simulink model "CodeMATLAB"  (R2020a)
settings: Solver=ode8  StartTime=0.0  StopTime=inf  FixedStep=0.05  RelTol=1e-3
PreLoadFcn:
  | waijung.modelPreload; % Required for working with Waijung Blockset. Do not remove.
undefined symbols (not defined in the file): Blocking, DiscIntNeverNeededParam, HSEOSC, LF, Link, LQFP100, Non, ST, STM32F407VG
libraries: amg_usbconverter_n_connect_lib x3, stm32f4_io_lib x2, simulink x2, stm32f4_tim_lib x1, stm32f4_reset_lib x1, stm32f4_device_config_lib x1
CloseFcn:
  | waijung.modelClose; % Required for working with Waijung Blockset. Do not remove.
settings Model: EnablePacing=on  Creator=tanda  LastModifiedBy=tanda
settings OptimizationCC: DefaultParameterBehavior=Inlined  EnhancedBackFolding=on  PassReuseOutputArgsAs=Individual arguments  ZeroExternalMemoryAtStartup=off  ZeroInternalMemoryAtStartup=off  OptimizeBlockOrder=speed  DifferentSizesBufferReuse=on  OptimizationCustomize=off  EfficientTunableParamExpr=on
settings DebuggingCC: ParameterTunabilityLossMsg=error
settings HardwareCC: ProdBitPerPointer=32  ProdBitPerSizeT=32  ProdBitPerPtrDiffT=32  ProdLargestAtomicFloat=None  ProdIntDivRoundTo=Undefined  ProdWordSize=32  ProdHWDeviceType=ARM Compatible->Cortex - M4  TargetEndianess=LittleEndian  TargetHWDeviceType=ARM Compatible->Cortex - M4
settings SFSimCC: MATLABDynamicMemAlloc=off
settings RTWCC: Description=STM32F4 Target  SystemTargetFile=stm32f4.tlc  GenerateMakefile=off  TemplateMakefile=ert_default_tmf
settings CodeAppCC: ForceParamTrailComments=on  IgnoreCustomStorageClasses=off  OperatorAnnotations=on  SimulinkDataObjDesc=on  SFDataObjDesc=on  InsertBlockDesc=on
settings STFCustomTargetCC: TargetLangStandard=C99 (ISO)  MultiwordLength=256  ModelReferenceCompliant=off  CombineOutputUpdateFcns=on  ERTCustomFileBanners=on  SupportContinuousTime=off  SupportNonInlinedSFcns=off  RemoveResetFunc=on  MATLABClassNameForMDSCustomization=Simulink.SoftwareTarget.ERTCustomization  SystemTargetFile=stm32f4.tlc
settings ERTTargetCC: TargetLangStandard=C99 (ISO)  ModelReferenceCompliant=off  ParMdlRefBuildCompliant=off  CompOptLevelCompliant=off  ConcurrentExecutionCompliant=off  ModelStepFunctionPrototypeControlCompliant=off  CPPClassGenCompliant=off  UseToolchainInfoCompliant=off  InlinedParameterPlacement=NonHierarchical  ERTSrcFileBannerTemplate=stm32f4_code_template.cgt  ERTHdrFileBannerTemplate=stm32f4_code_template.cgt  ERTDataSrcFileTemplate=stm32f4_code_template.cgt  ERTDataHdrFileTemplate=stm32f4_code_template.cgt  ERTCustomFileTemplate=stm32f4_file_process.tlc

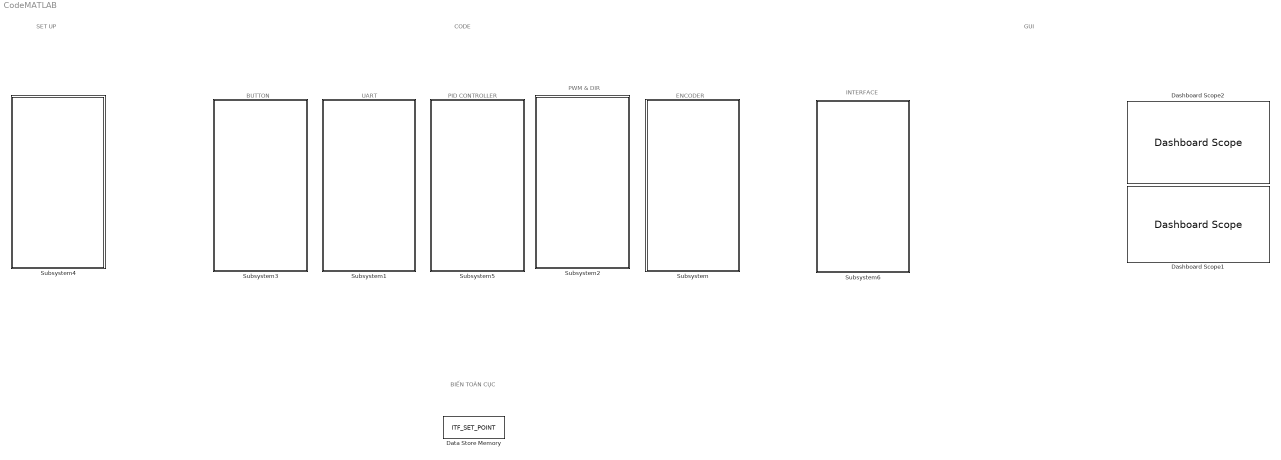
== system CodeMATLAB ==
  note: ENCODER
  note: SET UP
  note: CODE
  note: UART
  note: PWM & DIR
  note: BUTTON
  note: PID CONTROLLER
  note: INTERFACE
  note: GUI
  note: BIẾN TOÀN CỤC
  Dashboard Scope1 : DashboardScope
  Dashboard Scope2 : DashboardScope
  Data Store Memory : DataStoreMemory  DataStoreName=ITF_SET_POINT  ReadBeforeWriteMsg=warning  WriteAfterWriteMsg=warning  WriteAfterReadMsg=warning  ShowAdditionalParam=off  OutMin=-800  OutMax=800
      settings: DataLoggingMaxPoints=800
  Subsystem : Subsystem
  Subsystem1 : Subsystem
  Subsystem2 : Subsystem
  Subsystem3 : Subsystem
  Subsystem4 : Subsystem
  Subsystem5 : Subsystem
  Subsystem6 : Subsystem
  wires:
  ? -> ?

== system CodeMATLAB/Subsystem ==
  Doc encoder : Subsystem  TreatAsAtomicUnit=on
  Rate Transition2 : RateTransition  Deterministic=off  OutPortSampleTime=0.05
  Timer (Time Base) IRQ : stm32f4_tim_lib/Timer (Time Base) IRQ  configmode=Advance  timer=9  nvicprioritygroup=4  irqpreemptionpriority_g0=0  irqpreemptionpriority_g1=0  irqpreemptionpriority_g2=0  irqpreemptionpriority_g3=0  irqpreemptionpriority_g4=0  irqpreemptionpriority=0  irqsubpriority_g0=0  irqsubpriority_g1=0  irqsubpriority_g2=0  irqsubpriority_g3=0  irqsubpriority_g4=0  irqsubpriority=0  sampletime=0.05  autoreload=65115  prescaler=128  blockid=SubsystemTimerTimeBaseIRQ
      settings: SourceProductName=Waijung Blockset
  tag scope: SPEED=global
  wires:
  Doc encoder/1(Speed) -> Rate Transition2/1
  Timer (Time Base) IRQ/1 -> Doc encoder/Trigger
  Rate Transition2/1 -> [SPEED]

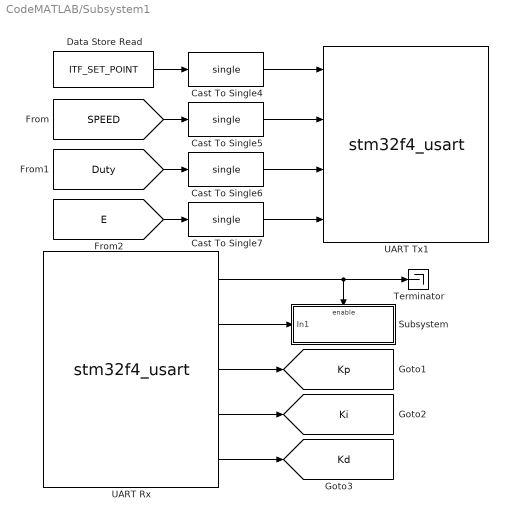
== system CodeMATLAB/Subsystem1 ==
  Cast To Single{4..7} (4 alike) : DataTypeConversion  OutDataTypeStr=single
  Data Store Read : DataStoreRead  DataStoreName=ITF_SET_POINT  DataStoreElements=ITF_SET_POINT
  Subsystem : Subsystem
  Terminator : Terminator
  UART Rx : S-Function  Priority=1  FunctionName=stm32f4_usart  Parameters=configuration,uartmodule,transfer,baudrate,inputtype,outputtype,confstr,binheaderarray,binterminatorarray,asciiheader,asciiterminator,bindatalength,packetmode,varname,sampletime,sampletimestr,blockid  SFunctionDeploymentMode=off  EnableBusSupport=off  mask(stm32f4_usart){configuration=Rx, uartmodule=6, baudrate=115200, databits=8, parity=No, stopbit=1, remaptxpin=Not used, remaprxpin=Not used, flowcontrol=None, remapctspin=Not used, remaprtspin=Not used, advanceoptions=off, rxbuffersize=512, txbuffersize=512, transfer=Non-Blocking, packetmode=Ascii, binheader='53', binterminator='00', porttype_double=0, porttype_single=0, porttype_int8=0, porttype_uint8=0, porttype_int16=0, porttype_uint16=0, porttype_int32=0, porttype_uint32=0, asciiformat='%f,%f,%f,%f', rx_asciiterminator=LF (0x0A - "\n"), tx_asciiterminator=LF (0x0A - "\n"), storagename=<empty>, varname=, inputtype=[0], outputtype=[5 3  1 1 1 1], binheaderarray=[0], binterminatorarray=[0], bindatalength=0, asciiheader='%f,%f,%f,%f\n', asciiterminator=[1 10], sampletime=-1, sampletimestr=-1, blockid=Subsystem1UARTRx, confstr=[ "dummy", "0", "*", "*", "0", "*", "*", "0", "*", "*", "0", "*", "*", "2", "5", "6", "2", "5", "1", "512", "512", "2", "6", "115200", "8", "No", "1", "None", "USART6"], lastmodule=1}
      mask prompts: uartmodule "UART Module"; baudrate "Baud rate (bps)"; databits "Data bits"; stopbit "Stop bit"; remaptxpin "Tx Pin"; remaprxpin "Rx Pin"; flowcontrol "Hardware flow control"; remapctspin "HW Flow control, CTS Pin"; remaprtspin "HW Flow control, RTS Pin"; advanceoptions "Advance options"; rxbuffersize "Rx buffer size (bytes)"; txbuffersize "Tx buffer size (bytes)"; packetmode "Packet mode"; binheader "Binary header (example: '7E 7E')"; binterminator "Binary terminator (example: '03 03')"; porttype_double "Number of data port, type DOUBLE"; porttype_single "Number of data port, type SINGLE"; porttype_int8 "Number of data port, type INT8"; porttype_uint8 "Number of data port, type UINT8"; porttype_int16 "Number of data port, type INT16"; porttype_uint16 "Number of data port, type UINT16"; porttype_int32 "Number of data port, type INT32"; porttype_uint32 "Number of data port, type UINT32"; asciiformat "Ascii format"; rx_asciiterminator "End of packet"; tx_asciiterminator "End of packet"; storagename "Buffer"; varname "Var name"; inputtype "Input data type"; outputtype "Output data type"; binheaderarray "Binary header"; binterminatorarray "Binary terminator"; bindatalength "Binary data length"; asciiheader "Ascii header (printf format)"; asciiterminator "Ascii terminator"; sampletime "Sample time (sec)"; sampletimestr "Compiled sample time (sec) in string"; confstr "Configuration string"; lastmodule "Last module selected"
      mask help:
      | Data type for Ascii format
      | %u, %i, %d, %o, %x: uint32
      | %e, %g, %f: single
      | %c: int8
      mask init:
      | stm32f4_usart_callback('init');
      mask Help: web(fullfile(waijungdocroot,'stm32f4_usart_rx.htm'), '-browser')
      mask TypeOptions configuration: Setup | Tx | Rx
      mask Callback configuration: stm32f4_usart_callback('configuration');
      mask TypeOptions uartmodule: 1 | 2 | 3 | 4 | 5 | 6
      mask Callback uartmodule: stm32f4_usart_callback('uartmodule');
      mask Callback baudrate: stm32f4_usart_callback('baudrate');
      mask TypeOptions databits: 8
      mask TypeOptions parity: No | Odd | Even
      mask TypeOptions stopbit: 0.5 | 1 | 1.5 | 2
      mask TypeOptions remaptxpin: Not used | A9 | B6
      mask TypeOptions remaprxpin: Not used | A10 | B7
      mask TypeOptions flowcontrol: None | RTS | CTS | RTS/CTS
      mask Callback flowcontrol: stm32f4_usart_callback('flowcontrol');
      mask TypeOptions remapctspin: Not used | A11
      mask TypeOptions remaprtspin: Not used | A12
      mask Callback advanceoptions: stm32f4_usart_callback('advanceoptions');
      mask TypeOptions rxbuffersize: 16 | 32 | 64 | 128 | 256 | 512 | 1024 | 2048
      mask TypeOptions txbuffersize: 16 | 32 | 64 | 128 | 256 | 512 | 1024 | 2048
      mask TypeOptions transfer: Blocking | Non-Blocking
      mask Callback transfer: stm32f4_usart_callback('transfer');
      mask TypeOptions packetmode: Ascii | Binary | Binary Vector | String Buffer | Raw Buffer | Read Line
      mask Callback packetmode: stm32f4_usart_callback('packetmode');
      mask Callback binheader: stm32f4_usart_callback('binheader');
      mask Callback binterminator: stm32f4_usart_callback('binterminator');
      mask Callback porttype_double: stm32f4_usart_callback('porttype');
      mask Callback porttype_single: stm32f4_usart_callback('porttype');
      mask Callback porttype_int8: stm32f4_usart_callback('porttype');
      mask Callback porttype_uint8: stm32f4_usart_callback('porttype');
      mask Callback porttype_int16: stm32f4_usart_callback('porttype');
      mask Callback porttype_uint16: stm32f4_usart_callback('porttype');
      mask Callback porttype_int32: stm32f4_usart_callback('porttype');
      mask Callback porttype_uint32: stm32f4_usart_callback('porttype');
      mask Callback asciiformat: stm32f4_usart_callback('asciiformat');
      mask TypeOptions rx_asciiterminator: CR (0x0D - "\r") | LF (0x0A - "\n") | CRLF (0x0D 0x0A - "\r\n")
      mask Callback rx_asciiterminator: stm32f4_usart_callback('rx_asciiterminator');
      mask TypeOptions tx_asciiterminator: CR (0x0D - "\r") | LF (0x0A - "\n") | CRLF (0x0D 0x0A - "\r\n") | None
      mask Callback tx_asciiterminator: stm32f4_usart_callback('tx_asciiterminator');
      mask TypeOptions storagename: <empty>
      mask Callback storagename: stm32f4_usart_callback('storagename');
      mask Callback varname: stm32f4_usart_callback('varname');
      mask Callback sampletime: stm32f4_usart_callback('sampletime');
      mask Callback sampletimestr: stm32f4_usart_callback('sampletimestr');
      mask Callback blockid: stm32f4_usart_callback('blockid');
      mask Display: text(0.05, 0.5, 'Module: USART6_Rx\nPacket: Ascii\nTransfer: Non-Blocking\nTs (sec): -1','ver','middle','hor','left'); port_label('output', 1,'READY'); port_label('output', 2,'single'); port_label('output', 3,'single'); port_label('output', 4,'single'); port_label('output', 5,'single');
  UART Tx1 : S-Function  Priority=1  FunctionName=stm32f4_usart  Parameters=configuration,uartmodule,transfer,baudrate,inputtype,outputtype,confstr,binheaderarray,binterminatorarray,asciiheader,asciiterminator,bindatalength,packetmode,varname,sampletime,sampletimestr,blockid  SFunctionDeploymentMode=off  EnableBusSupport=off  mask(stm32f4_usart){configuration=Tx, uartmodule=6, baudrate=115200, databits=8, parity=No, stopbit=1, remaptxpin=Not used, remaprxpin=Not used, flowcontrol=None, remapctspin=Not used, remaprtspin=Not used, advanceoptions=off, rxbuffersize=512, txbuffersize=512, transfer=Non-Blocking, packetmode=Ascii, binheader='7E 7E', binterminator='03 03', porttype_double=2, porttype_single=0, porttype_int8=0, porttype_uint8=0, porttype_int16=0, porttype_uint16=0, porttype_int32=0, porttype_uint32=0, asciiformat='%f,%f,%f,%f', rx_asciiterminator=CRLF (0x0D 0x0A - "\r\n"), tx_asciiterminator=LF (0x0A - "\n"), storagename=<empty>, varname=, inputtype=[4  1 1 1 1], outputtype=[0], binheaderarray=[0], binterminatorarray=[0], bindatalength=0, asciiheader='%f,%f,%f,%f\n', asciiterminator=[1 10], sampletime=0.05, sampletimestr=-1, blockid=Subsystem1UARTTx1, confstr=[ "dummy", "0", "*", "*", "0", "*", "*", "0", "*", "*", "0", "*", "*", "2", "5", "6", "2", "5", "1", "512", "512", "2", "6", "115200", "8", "No", "1", "None", "USART6"], lastmodule=1}
      mask prompts: uartmodule "UART Module"; baudrate "Baud rate (bps)"; databits "Data bits"; stopbit "Stop bit"; remaptxpin "Tx Pin"; remaprxpin "Rx Pin"; flowcontrol "Hardware flow control"; remapctspin "HW Flow control, CTS Pin"; remaprtspin "HW Flow control, RTS Pin"; advanceoptions "Advance options"; rxbuffersize "Rx buffer size (bytes)"; txbuffersize "Tx buffer size (bytes)"; packetmode "Packet mode"; binheader "Binary header (example: '7E 7E')"; binterminator "Binary terminator (example: '03 03')"; porttype_double "Number of data port, type DOUBLE"; porttype_single "Number of data port, type SINGLE"; porttype_int8 "Number of data port, type INT8"; porttype_uint8 "Number of data port, type UINT8"; porttype_int16 "Number of data port, type INT16"; porttype_uint16 "Number of data port, type UINT16"; porttype_int32 "Number of data port, type INT32"; porttype_uint32 "Number of data port, type UINT32"; asciiformat "Ascii format"; rx_asciiterminator "End of packet"; tx_asciiterminator "End of packet"; storagename "Buffer"; varname "Var name"; inputtype "Input data type"; outputtype "Output data type"; binheaderarray "Binary header"; binterminatorarray "Binary terminator"; bindatalength "Binary data length"; asciiheader "Ascii header (printf format)"; asciiterminator "Ascii terminator"; sampletime "Sample time (sec)"; sampletimestr "Compiled sample time (sec) in string"; confstr "Configuration string"; lastmodule "Last module selected"
      mask help:
      | Data type for Ascii format
      | %u, %i, %d, %o, %x: uint32
      | %e, %g, %f: single
      | %c: int8
      mask init:
      | stm32f4_usart_callback('init');
      mask Help: web(fullfile(waijungdocroot,'stm32f4_usart_tx.htm'), '-browser')
      mask TypeOptions configuration: Setup | Tx | Rx
      mask Callback configuration: stm32f4_usart_callback('configuration');
      mask TypeOptions uartmodule: 1 | 2 | 3 | 4 | 5 | 6
      mask Callback uartmodule: stm32f4_usart_callback('uartmodule');
      mask Callback baudrate: stm32f4_usart_callback('baudrate');
      mask TypeOptions databits: 8
      mask TypeOptions parity: No | Odd | Even
      mask TypeOptions stopbit: 0.5 | 1 | 1.5 | 2
      mask TypeOptions remaptxpin: Not used | A9 | B6
      mask TypeOptions remaprxpin: Not used | A10 | B7
      mask TypeOptions flowcontrol: None | RTS | CTS | RTS/CTS
      mask Callback flowcontrol: stm32f4_usart_callback('flowcontrol');
      mask TypeOptions remapctspin: Not used | A11
      mask TypeOptions remaprtspin: Not used | A12
      mask Callback advanceoptions: stm32f4_usart_callback('advanceoptions');
      mask TypeOptions rxbuffersize: 16 | 32 | 64 | 128 | 256 | 512 | 1024 | 2048
      mask TypeOptions txbuffersize: 16 | 32 | 64 | 128 | 256 | 512 | 1024 | 2048
      mask TypeOptions transfer: Blocking | Non-Blocking
      mask Callback transfer: stm32f4_usart_callback('transfer');
      mask TypeOptions packetmode: Ascii | Binary | Binary Vector | String Buffer | Raw Buffer
      mask Callback packetmode: stm32f4_usart_callback('packetmode');
      mask Callback binheader: stm32f4_usart_callback('binheader');
      mask Callback binterminator: stm32f4_usart_callback('binterminator');
      mask Callback porttype_double: stm32f4_usart_callback('porttype');
      mask Callback porttype_single: stm32f4_usart_callback('porttype');
      mask Callback porttype_int8: stm32f4_usart_callback('porttype');
      mask Callback porttype_uint8: stm32f4_usart_callback('porttype');
      mask Callback porttype_int16: stm32f4_usart_callback('porttype');
      mask Callback porttype_uint16: stm32f4_usart_callback('porttype');
      mask Callback porttype_int32: stm32f4_usart_callback('porttype');
      mask Callback porttype_uint32: stm32f4_usart_callback('porttype');
      mask Callback asciiformat: stm32f4_usart_callback('asciiformat');
      mask TypeOptions rx_asciiterminator: CR (0x0D - "\r") | LF (0x0A - "\n") | CRLF (0x0D 0x0A - "\r\n")
      mask Callback rx_asciiterminator: stm32f4_usart_callback('rx_asciiterminator');
      mask TypeOptions tx_asciiterminator: CR (0x0D - "\r") | LF (0x0A - "\n") | CRLF (0x0D 0x0A - "\r\n") | None
      mask Callback tx_asciiterminator: stm32f4_usart_callback('tx_asciiterminator');
      mask TypeOptions storagename: <empty>
      mask Callback storagename: stm32f4_usart_callback('storagename');
      mask Callback varname: stm32f4_usart_callback('varname');
      mask Callback sampletime: stm32f4_usart_callback('sampletime');
      mask Callback sampletimestr: stm32f4_usart_callback('sampletimestr');
      mask Callback blockid: stm32f4_usart_callback('blockid');
      mask Display: text(0.5, 0.5, 'Module: USART6_Tx\nPacket: Ascii\nTransfer: Non-Blocking\nTs (sec): -1','ver','middle','hor','center'); port_label('input', 1,'single'); port_label('input', 2,'single'); port_label('input', 3,'single'); port_label('input', 4,'single');
  tag scope: Kd=global, Ki=global, Kp=global
  wires:
  UART Rx/1 -> Terminator/1, Subsystem/Enable
  UART Rx/3 -> [Kp]
  UART Rx/4 -> [Ki]
  UART Rx/5 -> [Kd]
  Data Store Read/1 -> Cast To Single4/1
  [SPEED] -> Cast To Single5/1
  [Duty] -> Cast To Single6/1
  [E] -> Cast To Single7/1
  Cast To Single4/1 -> UART Tx1/1
  Cast To Single5/1 -> UART Tx1/2
  Cast To Single6/1 -> UART Tx1/3
  Cast To Single7/1 -> UART Tx1/4
  UART Rx/2 -> Subsystem/1(In1)

== system CodeMATLAB/Subsystem2 ==
  Xuat tin hieu : Subsystem
  wires:
  [Duty] -> Xuat tin hieu/1(Duty)

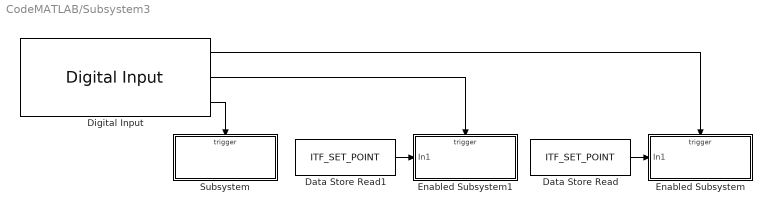
== system CodeMATLAB/Subsystem3 ==
  Data Store Read : DataStoreRead  DataStoreName=ITF_SET_POINT  DataStoreElements=ITF_SET_POINT
  Data Store Read1 : DataStoreRead  DataStoreName=ITF_SET_POINT  DataStoreElements=ITF_SET_POINT
  Digital Input : stm32f4_io_lib/Digital Input  port=D  speed=100  porttype=Pull Down  porttypestr=DOWN  use_pin0=on  use_pin1=off  use_pin2=on  use_pin3=off  use_pin4=on  use_pin5=off  use_pin6=off  use_pin7=off  use_pin8=off  use_pin9=off  use_pin10=off  use_pin11=off  use_pin12=off  use_pin13=off  use_pin14=off  use_pin15=off  pinstr=GPIO_Pin_0 | GPIO_Pin_2 | GPIO_Pin_4  usedpinarray="[1  0  1  0  1  0  0  0  0  0  0  0  0  0  0  0]"  bitbandingstr=|  sampletime=0.05  sampletimestr=-1  blockid=Subsystem3DigitalInput  enablecustomportlabel=off  glabalinit=off  cinputportlabel=In1, In2  coutputportlabel=Out1, Out2
      | #define Subsystem3DigitalInput_D0 Peripheral_BB(GPIOD->IDR, 0)  /* Output pin */
      | #define Subsystem3DigitalInput_D2 Peripheral_BB(GPIOD->IDR, 2)  /* Output pin */
      | #define Subsystem3DigitalInput_D4 Peripheral_BB(GPIOD->IDR, 4)  /* Output pin */
      settings: SourceProductName=Waijung Blockset
  Enabled Subsystem : Subsystem  TreatAsAtomicUnit=on
  Enabled Subsystem1 : Subsystem  TreatAsAtomicUnit=on
  Subsystem : Subsystem
  wires:
  Data Store Read1/1 -> Enabled Subsystem1/1(In1)
  Digital Input/1 -> Enabled Subsystem/Trigger
  Data Store Read/1 -> Enabled Subsystem/1(In1)
  Digital Input/2 -> Enabled Subsystem1/Trigger
  Digital Input/3 -> Subsystem/Trigger

== system CodeMATLAB/Subsystem4 ==
  Target Setup1 : stm32f4_device_config_lib/Target Setup  Priority=100  compiler=GNU ARM  previous_compiler=GNU ARM  mcu=STM32F407VG (LQFP100)  mcustr=STM32F407VG  clockconfig=HSEOSC-8MHz  system_stm32f4xx_c_path=C:\Users\tanda\OneDrive\Desktop\waijung18_11a\waijung_18.11a\targets\stm32f4_target\stm32f4\utils\system_stm32f4xx_default\STM32F40_41xxx\hseosc8mhz  showmemoryconfiguration=off  stacksize=0x2000  heapsize=0x2000  enableautocompiledownload=on  fullchiperase=on  programmerinterface=ST-Link  editctrlstr=on  compilercontrolstr=$(patsubst %, -I%, .) -mcpu=cortex-m4 -mthumb -mthumb-interwork -mfloat-abi=hard -mfpu=fpv4-sp-d16 -ffast-math -Wall -Wextra -Ofast  assemblercontrolstr=$(patsubst %, -I%, .) -mcpu=cortex-m4 -mthumb -mthumb-interwork -mfloat-abi=hard -mfpu=fpv4-sp-d16 -ffast-math -Wall -Wextra -Ofast -Wa,-amhls=$(<:.s=.lst) -D__STACK_SIZE=$(STACK_SIZE) -D__HEAP_SIZE=$(HEAP_SIZE)  linkercontrolstr=-T$(LD_SCRIPT) -g -Wl,-Map=$(MAP),--cref,--no-warn-mismatch -mcpu=cortex-m4 -mthumb -mthumb-interwork -mfloat-abi=hard -mfpu=fpv4-sp-d16 -specs=nosys.specs  runafterdownload=on  execprofile=None  profileruart=3  profilerbaud=500000  profilertxpin=D8  profilerinitstr=0.05,168000000,8400000,500000,0  manualsetsampletime=on  sampletime=0.05  blockid=Subsystem4TargetSetup1  systickreloadvalue=8400000  hseval=8000000  lastprofileruart=3  hclk=168000000  flashorigin=0x8000000  flashlength=1024k  ramorigin=0x20000000  ramlength=128k  useextram=off
      settings: SourceProductName=Waijung Blockset
  UART Setup1 : S-Function  Priority=1  FunctionName=stm32f4_usart  Parameters=configuration,uartmodule,transfer,baudrate,inputtype,outputtype,confstr,binheaderarray,binterminatorarray,asciiheader,asciiterminator,bindatalength,packetmode,varname,sampletime,sampletimestr,blockid  SFunctionDeploymentMode=off  EnableBusSupport=off  mask(stm32f4_usart){configuration=Setup, uartmodule=6, baudrate=115200, databits=8, parity=No, stopbit=1, remaptxpin=C6, remaprxpin=C7, flowcontrol=None, remapctspin=Not used, remaprtspin=Not used, advanceoptions=on, rxbuffersize=2048, txbuffersize=2048, transfer=Blocking, packetmode=Ascii, binheader='7E 7E', binterminator='03 03', porttype_double=1, porttype_single=0, porttype_int8=1, porttype_uint8=0, porttype_int16=0, porttype_uint16=0, porttype_int32=0, porttype_uint32=0, asciiformat='%d,%f', rx_asciiterminator=CRLF (0x0D 0x0A - "\r\n"), tx_asciiterminator=CR (0x0D - "\r"), storagename=<empty>, varname=, inputtype=[0], outputtype=[0], binheaderarray=[0], binterminatorarray=[0], bindatalength=0, asciiheader='', asciiterminator=[0], sampletime=-1, sampletimestr=-1, blockid=Subsystem4UARTSetup1, confstr=[ "dummy", "1", "C", "6", "1", "C", "7", "0", "*", "*", "0", "*", "*", "2", "5", "6", "2", "5", "1", "2048", "2048", "2", "6", "115200", "8", "No", "1", "None", "USART6"], lastmodule=6}
      mask prompts: uartmodule "UART Module"; baudrate "Baud rate (bps)"; databits "Data bits"; stopbit "Stop bit"; remaptxpin "Tx Pin"; remaprxpin "Rx Pin"; flowcontrol "Hardware flow control"; remapctspin "HW Flow control, CTS Pin"; remaprtspin "HW Flow control, RTS Pin"; advanceoptions "Advance options"; rxbuffersize "Rx buffer size (bytes)"; txbuffersize "Tx buffer size (bytes)"; packetmode "Packet mode"; binheader "Binary header (example: '7E 7E')"; binterminator "Binary terminator (example: '03 03')"; porttype_double "Number of data port, type DOUBLE"; porttype_single "Number of data port, type SINGLE"; porttype_int8 "Number of data port, type INT8"; porttype_uint8 "Number of data port, type UINT8"; porttype_int16 "Number of data port, type INT16"; porttype_uint16 "Number of data port, type UINT16"; porttype_int32 "Number of data port, type INT32"; porttype_uint32 "Number of data port, type UINT32"; asciiformat "Ascii format"; rx_asciiterminator "End of packet"; tx_asciiterminator "End of packet"; storagename "Buffer"; varname "Var name"; inputtype "Input data type"; outputtype "Output data type"; binheaderarray "Binary header"; binterminatorarray "Binary terminator"; bindatalength "Binary data length"; asciiheader "Ascii header (printf format)"; asciiterminator "Ascii terminator"; sampletime "Sample time (sec)"; sampletimestr "Compiled sample time (sec) in string"; confstr "Configuration string"; lastmodule "Last module selected"
      mask help:
      | Default STM32F4DISCOVERY + aMG F4 Connect 2 + aMG USB Converter N2 settings use
      |
      | USART3, Tx D8, Rx D9 and USB Serial Converter A.
      mask init:
      | stm32f4_usart_callback('init');
      mask Help: web(fullfile(waijungdocroot,'stm32f4_usart_setup.htm'), '-browser')
      mask TypeOptions configuration: Setup | Tx | Rx
      mask Callback configuration: stm32f4_usart_callback('configuration');
      mask TypeOptions uartmodule: 1 | 2 | 3 | 4 | 5 | 6
      mask Callback uartmodule: stm32f4_usart_callback('uartmodule');
      mask Callback baudrate: stm32f4_usart_callback('baudrate');
      mask TypeOptions databits: 8
      mask TypeOptions parity: No | Odd | Even
      mask TypeOptions stopbit: 0.5 | 1 | 1.5 | 2
      mask TypeOptions remaptxpin: Not used | C6
      mask TypeOptions remaprxpin: Not used | C7
      mask TypeOptions flowcontrol: None | RTS | CTS | RTS/CTS
      mask Callback flowcontrol: stm32f4_usart_callback('flowcontrol');
      mask TypeOptions remapctspin: Not used
      mask TypeOptions remaprtspin: Not used
      mask Callback advanceoptions: stm32f4_usart_callback('advanceoptions');
      mask TypeOptions rxbuffersize: 16 | 32 | 64 | 128 | 256 | 512 | 1024 | 2048
      mask TypeOptions txbuffersize: 16 | 32 | 64 | 128 | 256 | 512 | 1024 | 2048
      mask TypeOptions transfer: Blocking | Non-Blocking
      mask Callback transfer: stm32f4_usart_callback('transfer');
      mask TypeOptions packetmode: Ascii | Binary | String Buffer
      mask Callback packetmode: stm32f4_usart_callback('packetmode');
      mask Callback binheader: stm32f4_usart_callback('binheader');
      mask Callback binterminator: stm32f4_usart_callback('binterminator');
      mask Callback porttype_double: stm32f4_usart_callback('porttype');
      mask Callback porttype_single: stm32f4_usart_callback('porttype');
      mask Callback porttype_int8: stm32f4_usart_callback('porttype');
      mask Callback porttype_uint8: stm32f4_usart_callback('porttype');
      mask Callback porttype_int16: stm32f4_usart_callback('porttype');
      mask Callback porttype_uint16: stm32f4_usart_callback('porttype');
      mask Callback porttype_int32: stm32f4_usart_callback('porttype');
      mask Callback porttype_uint32: stm32f4_usart_callback('porttype');
      mask Callback asciiformat: stm32f4_usart_callback('asciiformat');
      mask TypeOptions rx_asciiterminator: CR (0x0D - "\r") | LF (0x0A - "\n") | CRLF (0x0D 0x0A - "\r\n")
      mask Callback rx_asciiterminator: stm32f4_usart_callback('rx_asciiterminator');
      mask TypeOptions tx_asciiterminator: CR (0x0D - "\r") | LF (0x0A - "\n") | CRLF (0x0D 0x0A - "\r\n") | None
      mask Callback tx_asciiterminator: stm32f4_usart_callback('tx_asciiterminator');
      mask TypeOptions storagename: <empty>
      mask Callback storagename: stm32f4_usart_callback('storagename');
      mask Callback varname: stm32f4_usart_callback('varname');
      mask Callback sampletime: stm32f4_usart_callback('sampletime');
      mask Callback sampletimestr: stm32f4_usart_callback('sampletimestr');
      mask Callback blockid: stm32f4_usart_callback('blockid');
      mask Display: text(0.5, 0.5, 'Module: USART6_Setup\nBaud (Bps): 115200\nDMA Buffer: 2048/2048\nTx/Rx Pin: C6/C7','ver','middle','hor','center');

== system CodeMATLAB/Subsystem5 ==
  Data Store Read : DataStoreRead  DataStoreName=ITF_SET_POINT
  PID : Subsystem
  tag scope: Duty=global
  wires:
  PID/1(Duty) -> [Duty]
  [SPEED] -> PID/2(Speed_present)
  Data Store Read/1 -> PID/1(Set speed)

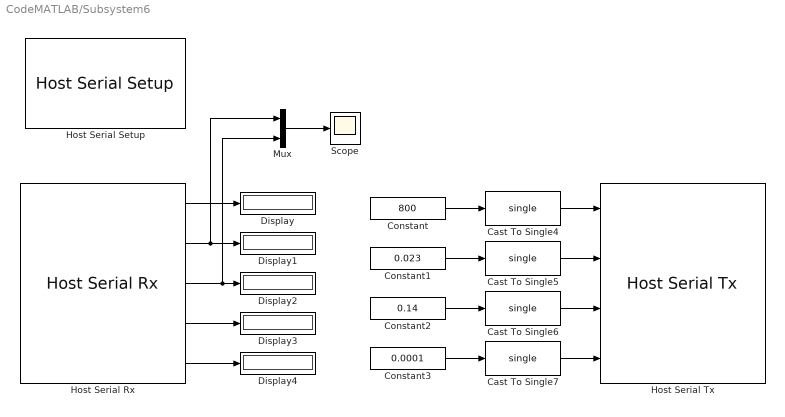
== system CodeMATLAB/Subsystem6 ==
  Cast To Single{4..7} (4 alike) : DataTypeConversion  OutDataTypeStr=single
  Constant : Constant  Value=800
  Constant1 : Constant  Value=0.023
  Constant2 : Constant  Value=0.14
  Constant3 : Constant  Value=0.0001
  Display{,1..4} (5 alike) : Display
  Host Serial Rx : amg_usbconverter_n_connect_lib/Host Serial Rx  conf=rx  port=COM3  baudrate=115200  databits=8  parity=None  stopbit=1  flowcontrol=None  transfer=Non-Blocking  timeout=5  packetmode=Ascii  enableinitialvalues=off  initialvalues=[]  binheader='53'  binterminator='00'  porttype_double=0  porttype_single=0  porttype_int8=0  porttype_uint8=40  porttype_int16=0  porttype_uint16=0  porttype_int32=0  porttype_uint32=0  asciiformat='%f,%f,%f,%f'  rx_asciiterminator="LF (0x0A - \"\\n\")"  tx_asciiterminator="CRLF (0x0D 0x0A - \"\\r\\n\")"  sampletime=-1  enablecustomportlabel=off  cinputportlabel=0  coutputportlabel=A  portpinstr=0  blockid=Subsystem6HostSerialRx  inputporttype=[]  inputportwidth=[]  inputportlabel={}  outputporttype=[3 1 1 1 1]  outputportwidth=[1 1 1 1 1]  outputportlabel={'READY','(single) %f','(single) %f','(single) %f','(single) %f'}  compat=0  optionstring="[\"Param1\",\"Param1\"]"  autoport='COM3'
      settings: SourceProductName=Waijung Blockset
  Host Serial Setup : amg_usbconverter_n_connect_lib/Host Serial Setup  conf=setup  port=COM3  baudrate=115200  databits=8  parity=None  stopbit=1  flowcontrol=None  transfer=Blocking  timeout=2  packetmode=Binary  initialvalues=[]  binheader='7E 7E'  binterminator='03 03'  porttype_double=0  porttype_single=1  porttype_int8=0  porttype_uint8=0  porttype_int16=0  porttype_uint16=0  porttype_int32=0  porttype_uint32=2  asciiformat='%d %u %x'  rx_asciiterminator="CRLF (0x0D 0x0A - \"\\r\\n\")"  tx_asciiterminator="CRLF (0x0D 0x0A - \"\\r\\n\")"  sampletime=-1  enablecustomportlabel=off  cinputportlabel=0  coutputportlabel=A  portpinstr=0  blockid=Subsystem6HostSerialSetup  inputporttype=[]  inputportwidth=[]  inputportlabel={}  outputporttype=[]  outputportwidth=[]  outputportlabel={}  compat=0  optionstring="[\"Param1\",\"Param1\"]"  autoport='COM3'
      settings: SourceProductName=Waijung Blockset
  Host Serial Tx : amg_usbconverter_n_connect_lib/Host Serial Tx  conf=tx  port=COM3  baudrate=115200  databits=8  parity=None  stopbit=1  flowcontrol=None  transfer=Blocking  timeout=2  packetmode=Ascii  initialvalues=[]  binheader='7E 7E'  binterminator='03 03'  porttype_double=0  porttype_single=0  porttype_int8=0  porttype_uint8=0  porttype_int16=0  porttype_uint16=0  porttype_int32=0  porttype_uint32=2  asciiformat='%f,%f,%f,%f'  rx_asciiterminator="CRLF (0x0D 0x0A - \"\\r\\n\")"  tx_asciiterminator="LF (0x0A - \"\\n\")"  sampletime=-1  enablecustomportlabel=off  cinputportlabel=0  coutputportlabel=A  portpinstr=0  blockid=Subsystem6HostSerialTx  inputporttype=[1 1 1 1]  inputportwidth=[1 1 1 1]  inputportlabel={'%f (single)','%f (single)','%f (single)','%f (single)'}  outputporttype=[]  outputportwidth=[]  outputportlabel={}  compat=0  optionstring="[\"Param1\",\"Param1\"]"  autoport='COM3'
      settings: SourceProductName=Waijung Blockset
  Mux : Mux  Inputs=2
  Scope : Scope
  wires:
  Cast To Single7/1 -> Host Serial Tx/4
  Cast To Single6/1 -> Host Serial Tx/3
  Cast To Single5/1 -> Host Serial Tx/2
  Constant2/1 -> Cast To Single6/1
  Constant1/1 -> Cast To Single5/1
  Host Serial Rx/2 -> Mux/1, Display1/1
  Host Serial Rx/5 -> Display4/1
  Host Serial Rx/3 -> Mux/2, Display2/1
  Host Serial Rx/1 -> Display/1
  Constant/1 -> Cast To Single4/1
  Constant3/1 -> Cast To Single7/1
  Cast To Single4/1 -> Host Serial Tx/1
  Host Serial Rx/4 -> Display3/1
  Mux/1 -> Scope/1

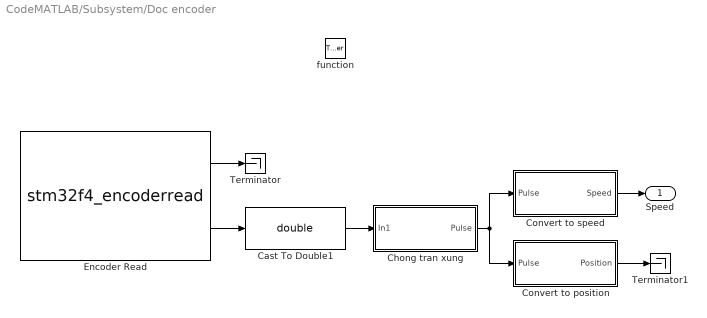
== system CodeMATLAB/Subsystem/Doc encoder ==
  function : TriggerPort  TriggerType=function-call  VariantControl=Variant
  Cast To Double1 : DataTypeConversion  OutDataTypeStr=double
  Chong tran xung : Subsystem
  Convert to position : Subsystem
  Convert to speed : Subsystem
  Encoder Read : S-Function  FunctionName=stm32f4_encoderread  Parameters=sampletime,sampletimestr,blockid,timer,apb,portstr,pinstr,pinmat,chmat,filterstr,filter,factor,rstcnt,ppr  SFunctionDeploymentMode=off  EnableBusSupport=off  mask(stm32f4_encoderread){timer=1, ch1=E9, ch2=E11, ppr=0, rstcnt=off, filterstr=No filter; sampling is done at fDTS, sampletime=-1, sampletimestr=-1, blockid=SubsystemDocencoderEncoderRead, absresetinput=off, portpinstr=E9,E11, portstr=["E"], pinstr=["GPIO_Pin_9 | GPIO_Pin_11"], pinmat=[2 9 11], chmat=[1  2], apb=2, filter=0, factor=4}
      mask prompts: ch1 "Channel A Input Pin"; ch2 "Channel B Input Pin"; ppr "PPR (Number of pulses generated per revolution)"; rstcnt "Reset counter after every counter read"; filterstr "Built-in Input Capture Filter"; sampletime "Sample time (sec)"; sampletimestr "Compiled sample time (sec) in string"; absresetinput "Enable absolute position reset input signal"; portpinstr "Port pin string"; portstr "Port string"; pinstr "Pin string"; pinmat "Pin matrix"; chmat "Channel order"; filter "Filter ID"
      mask help:
      | The output Direction (uint32) is the direction of rotation either 0 or 1.
      |
      | The output Position (count) (uint32) is the count of number of edges of the encoder output signals from either channel A and B. The decoder is set to count at every rising and falling edge of both channel A and B (4x) or (x2) for one channel. For example, if an encoder has 180 pulses per revolution (PPS) and two channels are selected, the maximum count is 720 per revolution (4x180 = 720), i.e. from 0 to 719.
      mask init:
      | stm32f4_encoderread_callback('init');
      mask Help: web(fullfile(waijungdocroot,'stm32f4_encoderread.htm'),'-browser')
      mask TypeOptions timer: 1 | 2 | 3 | 4 | 5 | 8
      mask Callback timer: stm32f4_encoderread_callback('timer');
      mask TypeOptions ch1: Not available - Do not use | E9 | A8
      mask Callback ch1: stm32f4_encoderread_callback('chA');
      mask TypeOptions ch2: Not available - Do not use | E11 | A9
      mask Callback ch2: stm32f4_encoderread_callback('chB');
      mask Callback ppr: stm32f4_encoderread_callback('ppr');
      mask Callback rstcnt: stm32f4_encoderread_callback('rstcnt');
      mask TypeOptions filterstr: No filter; sampling is done at fDTS | fSAMPLING=fCK_INT; N=2 | fSAMPLING=fCK_INT; N=4 | fSAMPLING=fCK_INT; N=8 | fSAMPLING=fDTS/2; N=6 | fSAMPLING=fDTS/2; N=8 | fSAMPLING=fDTS/4; N=6 | fSAMPLING=fDTS/4; N=8 | fSAMPLING=fDTS/8; N=6 | fSAMPLING=fDTS/8; N=8 | fSAMPLING=fDTS/16; N=5 | fSAMPLING=fDTS/16; N=6 | fSAMPLING=fDTS/16; N=8 | fSAMPLING=fDTS/32; N=5 | fSAMPLING=fDTS/32; N=6 | fSAMPLING=fDTS/32; N=8
      mask Callback filterstr: stm32f4_encoderread_callback('filterstr');
      mask Callback sampletimestr: stm32f4_encoderread_callback('sampletimestr');
      mask Callback blockid: stm32f4_encoderread_callback('blockid');
      mask Display: text(0.05, 0.5, 'Timer: 1\nInput pins [CH_A, CH_B]: [E9,E11]\nRST Counter: No\nTs (sec): -1','ver','middle','hor','left');port_label('output', 1, 'Direction');port_label('output', 2, 'Position (count)')
  Terminator : Terminator
  Terminator1 : Terminator
  Speed : Outport
  wires:
  Encoder Read/2 -> Cast To Double1/1
  Cast To Double1/1 -> Chong tran xung/1(In1)
  Encoder Read/1 -> Terminator/1
  Chong tran xung/1(Pulse) -> Convert to position/1(Pulse), Convert to speed/1(Pulse)
  Convert to speed/1(Speed) -> Speed/1
  Convert to position/1(Position) -> Terminator1/1

== system CodeMATLAB/Subsystem1/Subsystem ==
  In1 : Inport
  Enable : EnablePort
  Data Store Write : DataStoreWrite  DataStoreName=ITF_SET_POINT  DataStoreElements=ITF_SET_POINT
  wires:
  In1/1 -> Data Store Write/1

== system CodeMATLAB/Subsystem2/Xuat tin hieu ==
  Duty : Inport  OutDataTypeStr=double
  Basic PWM : S-Function  FunctionName=stm32f4_basicpwm  Parameters=timer,pwmperiod,ch1pin,ch2pin,ch3pin,ch4pin,sampletime,sampletimestr,blockid,apb,portstr,pinstr,pinmat,timarr,timprescale,chmat,polaritystr  SFunctionDeploymentMode=off  EnableBusSupport=off  mask(stm32f4_basicpwm){timer=2, pwmperiod=0.0001, polarity=Active Low, polaritystr=TIM_OCPolarity_Low, ch1pin=Not available - Do not use, ch2pin=Not available - Do not use, ch3pin=A2, ch4pin=Not available - Do not use, sampletime=0.05, sampletimestr=-1, blockid=Subsystem2XuattinhieuBasicPWM, portpinstr=,,A2,, enablecustomportlabel=off, cinputportlabel=In1, In2, In3, In4, coutputportlabel=0, apb=1, portstr=["A"], pinstr=["GPIO_Pin_2"], pinmat=[1 2], timarr=8399, timprescale=0, chmat=[3]}
      mask prompts: pwmperiod "PWM Period (seconds)"; ch1pin "Channel 1"; ch2pin "Channel 2"; ch3pin "Channel 3"; ch4pin "Channel 4"; sampletime "Sample time (sec)"; sampletimestr "Compiled sample time (sec) in string"; portpinstr "Port pin string"; enablecustomportlabel "Enable custom port labels"; cinputportlabel "Custom input port labels (Ex. In1, In2, In3)"; coutputportlabel "Custom output port labels (Ex. Out1, Out2, Out3)"; portstr "Port string"; pinstr "Pin string"; pinmat "Pin matrix"; timarr "Timer ARR"; timprescale "Timer PRESCALE"; chmat "Channel order"
      mask help:
      | This block implements basic Edge-aligned Pulse Width Modulation (PWM) generation.
      | All timers are 16-bit. The PWM period is fixed (per timer).
      mask init:
      | stm32f4_basicpwm_callback('init');
      mask Help: web(fullfile(waijungdocroot,'stm32f4_basicpwm.htm'),'-browser')
      mask TypeOptions timer: 1 | 2 | 3 | 4 | 5 | 8 | 9 | 10 | 11 | 12 | 13 | 14
      mask Callback timer: stm32f4_basicpwm_callback('timer');
      mask Callback pwmperiod: stm32f4_basicpwm_callback('pwmperiod');
      mask TypeOptions polarity: Active High | Active Low
      mask Callback polarity: stm32f4_basicpwm_callback('polarity');
      mask TypeOptions ch1pin: Not available - Do not use | A0 | A5 | A15
      mask Callback ch1pin: stm32f4_basicpwm_callback('ch1pin');
      mask TypeOptions ch2pin: Not available - Do not use | A1 | B3
      mask Callback ch2pin: stm32f4_basicpwm_callback('ch2pin');
      mask TypeOptions ch3pin: Not available - Do not use | A2 | B10
      mask Callback ch3pin: stm32f4_basicpwm_callback('ch3pin');
      mask TypeOptions ch4pin: Not available - Do not use | A3 | B11
      mask Callback ch4pin: stm32f4_basicpwm_callback('ch4pin');
      mask Callback sampletime: stm32f4_basicpwm_callback('sampletime');
      mask Callback sampletimestr: stm32f4_basicpwm_callback('sampletimestr');
      mask Callback blockid: stm32f4_basicpwm_callback('blockid');
      mask Callback enablecustomportlabel: stm32f4_basicpwm_callback('enablecustomportlabel');
      mask Display: text(0.95, 0.5, 'Timer: 2\nPolarity: Active Low\nPeriod (sec) 0.0001\nTs (sec): -1','ver','middle','hor','right');port_label('input', 1,'CH3 (A2)')
  Digital Output : stm32f4_io_lib/Digital Output  use_bitband=on  port=A  speed=100  porttype=Push Pull  porttypestr=PP  use_pin0=off  use_pin1=off  use_pin2=off  use_pin3=off  use_pin4=on  use_pin5=off  use_pin6=off  use_pin7=off  use_pin8=off  use_pin9=off  use_pin10=off  use_pin11=off  use_pin12=off  use_pin13=off  use_pin14=off  use_pin15=off  pinstr=GPIO_Pin_4  usedpinarray="[0  0  0  0  1  0  0  0  0  0  0  0  0  0  0  0]"  bitbandingstr="#define Subsystem2XuattinhieuDigitalOutput_A4 Peripheral_BB(GPIOA->ODR, 4)  /* Output pin */"  sampletime=0.05  sampletimestr=-1  blockid=Subsystem2XuattinhieuDigitalOutput  enablecustomportlabel=off  globalinit=off  cinputportlabel=In1, In2  coutputportlabel=0
      settings: SourceProductName=Waijung Blockset
  MATLAB Function : MATLAB Function  TreatAsAtomicUnit=on
  wires:
  MATLAB Function/1(PWM) -> Basic PWM/1
  MATLAB Function/2(Dir) -> Digital Output/1
  Duty/1 -> MATLAB Function/1(Duty)

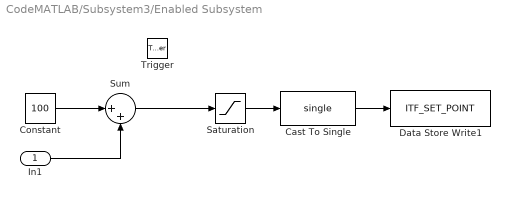
== system CodeMATLAB/Subsystem3/Enabled Subsystem ==
  In1 : Inport
  Trigger : TriggerPort  VariantControl=Variant  PortDimensions=1
  Cast To Single : DataTypeConversion  OutDataTypeStr=single
  Constant : Constant  Value=100
  Data Store Write1 : DataStoreWrite  DataStoreName=ITF_SET_POINT  DataStoreElements=ITF_SET_POINT
  Saturation : Saturate  UpperLimit=800  LowerLimit=-800
  Sum : Sum  Inputs=|++
  wires:
  Constant/1 -> Sum/1
  Sum/1 -> Saturation/1
  In1/1 -> Sum/2
  Saturation/1 -> Cast To Single/1
  Cast To Single/1 -> Data Store Write1/1

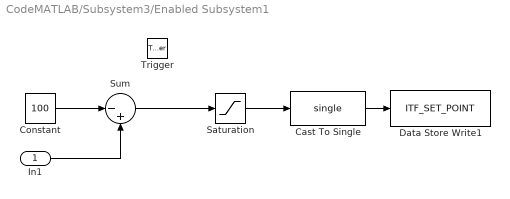
== system CodeMATLAB/Subsystem3/Enabled Subsystem1 ==
  In1 : Inport
  Trigger : TriggerPort  VariantControl=Variant  InitialTriggerSignalState=zero  PortDimensions=1
  Cast To Single : DataTypeConversion  OutDataTypeStr=single
  Constant : Constant  Value=100
  Data Store Write1 : DataStoreWrite  DataStoreName=ITF_SET_POINT  DataStoreElements=ITF_SET_POINT
  Saturation : Saturate  UpperLimit=800  LowerLimit=-800
  Sum : Sum  Inputs=|-+
  wires:
  Constant/1 -> Sum/1
  Sum/1 -> Saturation/1
  Saturation/1 -> Cast To Single/1
  In1/1 -> Sum/2
  Cast To Single/1 -> Data Store Write1/1

== system CodeMATLAB/Subsystem3/Subsystem ==
  Trigger : TriggerPort  VariantControl=Variant  InitialTriggerSignalState=zero  PortDimensions=1
  System Reset : stm32f4_reset_lib/System Reset  conf=<empty>  sampletime=-1  sampletimestr=-1  blockid=Subsystem3SubsystemSystemReset  inputarray=[]  inputlabelarray={}  outputarray=[]  outputlabelarray={}  compat=0  confstr="[\"Param1\",\"Param1\"]"
      settings: SourceProductName=Waijung Blockset

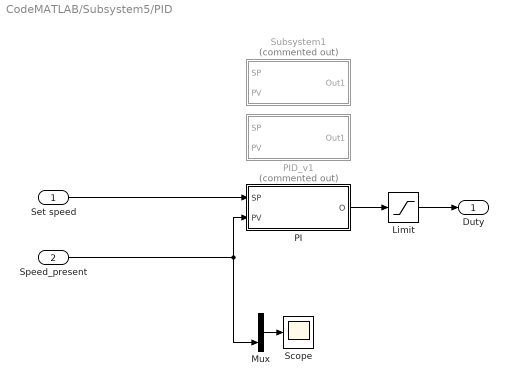
== system CodeMATLAB/Subsystem5/PID ==
  Set speed : Inport
  Speed_present : Inport  Port=2
  Limit : Saturate  UpperLimit=95  LowerLimit=-95
  Mux : Mux  Inputs=2
  PI : Subsystem
  PID_v1 : Subsystem  Commented=on
  Scope : Scope
  Subsystem1 : Subsystem  Commented=on
  Duty : Outport
  wires:
  Limit/1 -> Duty/1
  PI/1(O) -> Limit/1
  Mux/1 -> Scope/1
  Speed_present/1 -> PI/2(PV), Mux/2
  Set speed/1 -> PI/1(SP)

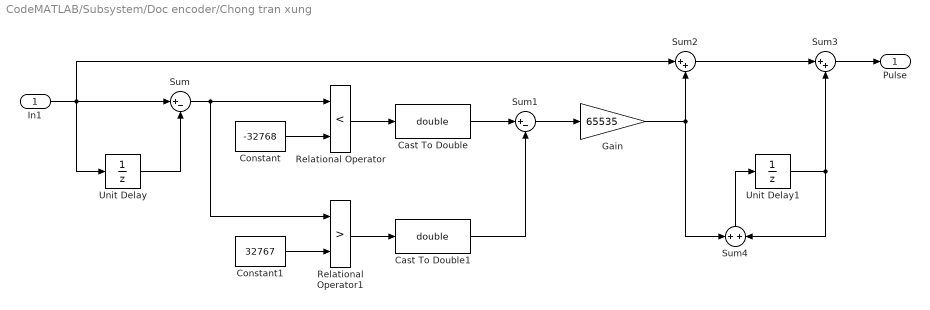
== system CodeMATLAB/Subsystem/Doc encoder/Chong tran xung ==
  In1 : Inport
  Cast To Double : DataTypeConversion  OutDataTypeStr=double
  Cast To Double1 : DataTypeConversion  OutDataTypeStr=double
  Constant : Constant  Value=-32768
  Constant1 : Constant  Value=32767
  Gain : Gain  Gain=65535
  Relational Operator : RelationalOperator  Operator=<  OutDataTypeStr=boolean  RndMeth=Simplest
  Relational Operator1 : RelationalOperator  Operator=>  OutDataTypeStr=boolean  RndMeth=Simplest
  Sum : Sum  Inputs=|+-
  Sum1 : Sum  Inputs=|+-
  Sum2 : Sum  Inputs=|++
  Sum3 : Sum  Inputs=|++
  Sum4 : Sum  Inputs=+|+
  Unit Delay : UnitDelay  SampleTime=-1  HasFrameUpgradeWarning=on
  Unit Delay1 : UnitDelay  SampleTime=-1  HasFrameUpgradeWarning=on
  Pulse : Outport
  wires:
  Sum/1 -> Relational Operator/1, Relational Operator1/1
  Relational Operator/1 -> Cast To Double/1
  Cast To Double/1 -> Sum1/1
  Sum1/1 -> Gain/1
  Unit Delay/1 -> Sum/2
  In1/1 -> Sum2/1, Unit Delay/1, Sum/1
  Constant/1 -> Relational Operator/2
  Constant1/1 -> Relational Operator1/2
  Relational Operator1/1 -> Cast To Double1/1
  Cast To Double1/1 -> Sum1/2
  Sum2/1 -> Sum3/1
  Unit Delay1/1 -> Sum4/2, Sum3/2
  Gain/1 -> Sum4/1, Sum2/2
  Sum4/1 -> Unit Delay1/1
  Sum3/1 -> Pulse/1

== system CodeMATLAB/Subsystem/Doc encoder/Convert to position ==
  Pulse : Inport
  Angle : Gain  Gain=360/800
  Position : Outport
  wires:
  Pulse/1 -> Angle/1
  Angle/1 -> Position/1

== system CodeMATLAB/Subsystem/Doc encoder/Convert to speed ==
  Pulse : Inport
  PPM : Gain  Gain=60/(0.05*800)  OutDataTypeStr=double
  Sum1 : Sum  Inputs=|+-  OutDataTypeStr=double
  Unit Delay1 : UnitDelay  SampleTime=-1  HasFrameUpgradeWarning=on
  Speed : Outport
  wires:
  PPM/1 -> Speed/1
  Sum1/1 -> PPM/1
  Pulse/1 -> Unit Delay1/1, Sum1/1
  Unit Delay1/1 -> Sum1/2

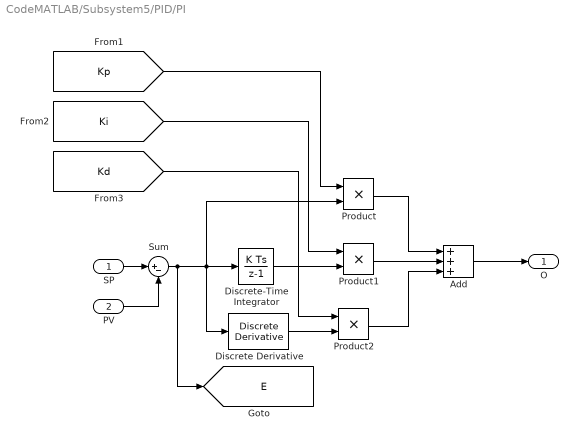
== system CodeMATLAB/Subsystem5/PID/PI ==
  SP : Inport
  PV : Inport  Port=2
  Add : Sum  Inputs=+++
  Discrete Derivative : simulink/Discrete/Discrete Derivative  gainval=1.0  ICPrevScaledInput=0.0  OutMin=[]  OutMax=[]  OutDataType=fixdt(1, 16)  OutScaling=2^-10  DoSatur=off
  Discrete-Time Integrator : DiscreteIntegrator  SampleTime=0.1  ICPrevOutput=DiscIntNeverNeededParam  ICPrevScaledInput=DiscIntNeverNeededParam
  Product : Product
  Product1 : Product
  Product2 : Product
  Sum : Sum  Inputs=|+-
  O : Outport
  tag scope: E=global
  wires:
  Add/1 -> O/1
  Product1/1 -> Add/2
  Discrete-Time Integrator/1 -> Product1/2
  Discrete Derivative/1 -> Product2/2
  Product2/1 -> Add/3
  Product/1 -> Add/1
  SP/1 -> Sum/1
  PV/1 -> Sum/2
  [Kp] -> Product/1
  [Ki] -> Product1/1
  [Kd] -> Product2/1
  Sum/1 -> [E], Product/2, Discrete Derivative/1, Discrete-Time Integrator/1

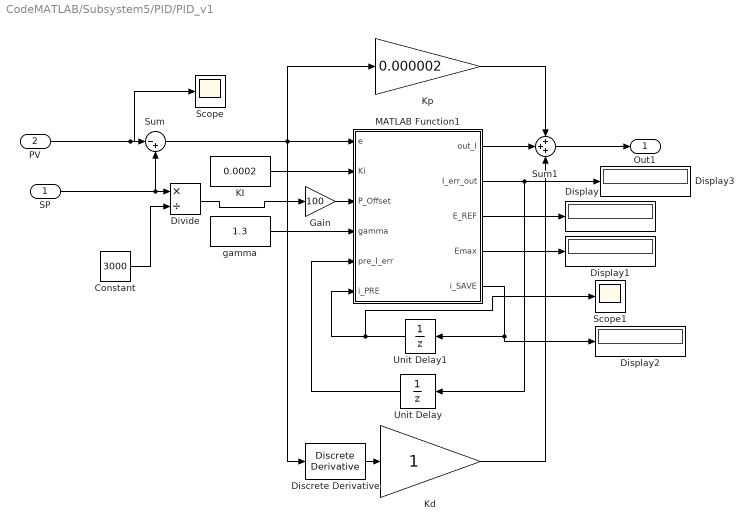
== system CodeMATLAB/Subsystem5/PID/PID_v1 ==
  SP : Inport
  PV : Inport  Port=2
  Constant : Constant  Value=3000
  Discrete Derivative : simulink/Discrete/Discrete Derivative  gainval=1.0  ICPrevScaledInput=0.0  OutMin=[]  OutMax=[]  OutDataType=fixdt(1, 16)  OutScaling=2^-10  DoSatur=off
  Display{,1..3} (4 alike) : Display
  Divide : Product  Inputs=*/
  Gain : Gain  Gain=100
  KI : Constant  Value=0.0002
  Kd : Gain
  Kp : Gain  Gain=0.000002
  MATLAB Function1 : MATLAB Function  TreatAsAtomicUnit=on
  Scope : Scope
  Scope1 : Scope
  Sum : Sum  Inputs=|-+
  Sum1 : Sum  Inputs=+++
  Unit Delay : UnitDelay  SampleTime=0.05  HasFrameUpgradeWarning=on
  Unit Delay1 : UnitDelay  SampleTime=0.05  HasFrameUpgradeWarning=on
  gamma : Constant  Value=1.3
  Out1 : Outport
  wires:
  gamma/1 -> MATLAB Function1/4(gamma)
  Unit Delay1/1 -> Scope1/1, MATLAB Function1/6(i_PRE)
  Kd/1 -> Sum1/3
  MATLAB Function1/1(out_I) -> Sum1/2
  Unit Delay/1 -> MATLAB Function1/5(pre_I_err)
  PV/1 -> Scope/1, Sum/1
  Sum1/1 -> Out1/1
  Kp/1 -> Sum1/1
  Discrete Derivative/1 -> Kd/1
  KI/1 -> MATLAB Function1/2(Ki)
  MATLAB Function1/2(I_err_out) -> Display3/1, Unit Delay/1
  SP/1 -> Sum/2, Divide/1
  Sum/1 -> Discrete Derivative/1, Kp/1, MATLAB Function1/1(e)
  Constant/1 -> Divide/2
  Divide/1 -> Gain/1
  MATLAB Function1/3(E_REF) -> Display/1
  MATLAB Function1/4(Emax) -> Display1/1
  Gain/1 -> MATLAB Function1/3(P_Offset)
  MATLAB Function1/5(i_SAVE) -> Display2/1, Unit Delay1/1

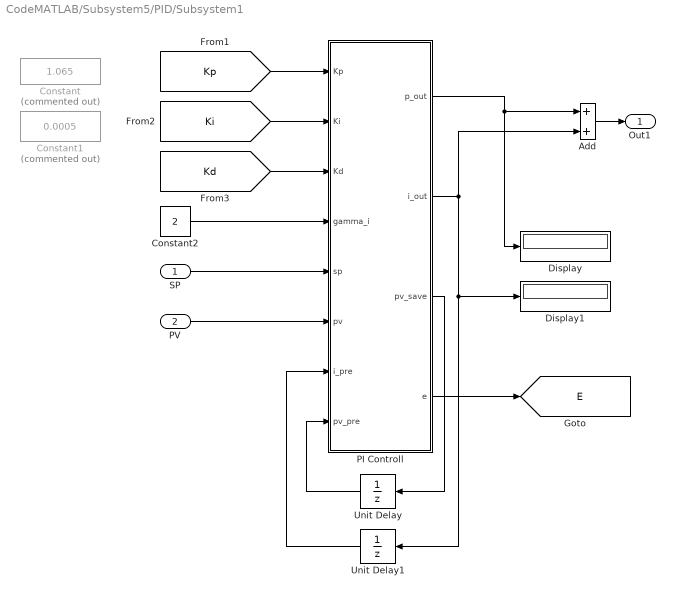
== system CodeMATLAB/Subsystem5/PID/Subsystem1 ==
  SP : Inport
  PV : Inport  Port=2
  Add : Sum
  Constant : Constant  Commented=on  Value=1.065
  Constant1 : Constant  Commented=on  Value=0.0005
  Constant2 : Constant  Value=2
  Display : Display
  Display1 : Display
  PI Controll : MATLAB Function  TreatAsAtomicUnit=on
  Unit Delay : UnitDelay  SampleTime=-1  HasFrameUpgradeWarning=on
  Unit Delay1 : UnitDelay  SampleTime=-1  HasFrameUpgradeWarning=on
  Out1 : Outport
  tag scope: E=global
  wires:
  SP/1 -> PI Controll/5(sp)
  PV/1 -> PI Controll/6(pv)
  PI Controll/3(pv_save) -> Unit Delay/1
  Unit Delay/1 -> PI Controll/8(pv_pre)
  PI Controll/1(p_out) -> Display/1, Add/1
  Unit Delay1/1 -> PI Controll/7(i_pre)
  Add/1 -> Out1/1
  PI Controll/2(i_out) -> Unit Delay1/1, Display1/1, Add/2
  Constant2/1 -> PI Controll/4(gamma_i)
  [Kd] -> PI Controll/3(Kd)
  PI Controll/4(e) -> [E]
  [Kp] -> PI Controll/1(Kp)
  [Ki] -> PI Controll/2(Ki)

== matlab function CodeMATLAB/Subsystem5/PID/PID_v1/MATLAB Function1 ==
  data: out_I output; e input; Ki input; P_Offset input; gamma input; pre_I_err input; I_err_out output; E_REF output; Emax output; i_SAVE output; i_PRE input
function [out_I,I_err_out,E_REF,Emax,i_SAVE]= fcn(e,Ki,P_Offset,gamma,pre_I_err,i_PRE)
    dt=0.05;
    E_REF = P_Offset/(Ki*dt);
    Emax = E_REF*gamma;
%     i_SAVE = i_PRE +1;
    if(i_PRE > 0)
        % 2st loop and so on      
        if(e<100)
            I_err_out = e + pre_I_err;
        else
            I_err_out = pre_I_err;
        end
            i_SAVE = i_PRE;
    else
        % 1st loop
        I_err_out = E_REF;
        i_SAVE=1;
    end
    
    
    
    if(I_err_out>Emax)
        I_err_out = Emax;
    end
    if(I_err_out<-Emax)
        I_err_out = - Emax;
    end
    
    out_I = Ki * I_err_out * dt;          %% [0 1]
        
end

== matlab function CodeMATLAB/Subsystem2/Xuat tin hieu/MATLAB Function ==
  data: Duty input; PWM output; Dir output
function [PWM,Dir] = fcn(Duty)
    if(Duty>=0)
        Dir=1;
        PWM=Duty;
    else
        PWM= -Duty;
        Dir=0;
    end
end

== matlab function CodeMATLAB/Subsystem5/PID/Subsystem1/PI Controll ==
  data: Kp input; Ki input; Kd input; gamma_i input; p_out output; i_out output; sp input; pv input; i_pre input; pv_pre input; pv_save output; e output
function [p_out,i_out,pv_save,e] = fcn(Kp,Ki,Kd,gamma_i,sp,pv,i_pre,pv_pre)
persistent k

if(isempty(k))
    k = 0;
end

e=sp-pv;
pv_save=pv; 
if(abs(sp)>500)
    %% SP 500-800
    p_out=Kp*1*(sp/1521)*50;
    if(abs(e)<(0.1*abs(sp)))
    i_out=i_pre+Ki*e*0.015;
    else
    i_out=i_pre;
    end
    if(i_out>gamma_i)
     i_out=gamma_i;
    end
    if(i_out<-gamma_i)
     i_out=-gamma_i;
    end
elseif(abs(sp)>200&&abs(sp)<600)
    %% SP 300-500
    p_out=Kp*(sp/550)*20;
    if(abs(e)<(0.2*abs(sp)))
    i_out=i_pre+Ki*e*0.025;
    else
    i_out=i_pre;
    end
    if(i_out>gamma_i)
     i_out=gamma_i;
    end
    if(i_out<-gamma_i)
     i_out=-gamma_i;
    end
else
    %% SP 200
    if(abs(sp) == 200)
    p_out=Kp*1.1*(sp/350)*15;
    if(abs(e)<(1*abs(sp)))
    i_out=i_pre+Ki*e*0.015;
    else
    i_out=i_pre;
    end
    if(i_out>gamma_i)
     i_out=gamma_i;
    end
    if(i_out<-gamma_i)
     i_out=-gamma_i;
    end
    else
    %% SP 100  
    p_out=Kp*(sp/130)*8;
    i_out=i_pre+Ki*e*0.01;
    if(i_out>gamma_i)
     i_out=gamma_i;
    end
    if(i_out<-gamma_i)
     i_out=-gamma_i;
    end
end
end
